simulink model "PMSMfoc_SVPWM"  (R2021b)
settings: Solver=ode3  StartTime=0.0  StopTime=0.3  FixedStep=1e-6  RelTol=1e-3
libraries: simulink x6, slpidlib x3, dsparch4 x3, spsDCVoltageSourceLib x1, spsPermanentMagnetSynchronousMachineLib x1, spsSVPWMGenerator2LevelLib x1, spsabctoAlphaBetaZeroLib x1, spsabctodq0Lib x1, spsdq0toAlphaBetaZeroLib x1, spspowerguiLib x1, spsUniversalBridgeLib x1
settings Model: Creator=zyh  LastModifiedBy=zyh
settings SolverCC: AlgebraicLoopSolver=TrustRegion
settings DataIOCC: ReturnWorkspaceOutputs=off
settings DebuggingCC: MaskedZcDiagnostic=none  IgnoredZcDiagnostic=none  SFMachineParentedDataDiag=warning  ArithmeticOperatorsInVariantConditions=warning
settings SFSimCC: CustomCodeUndefinedFunction=UseInterfaceOnly

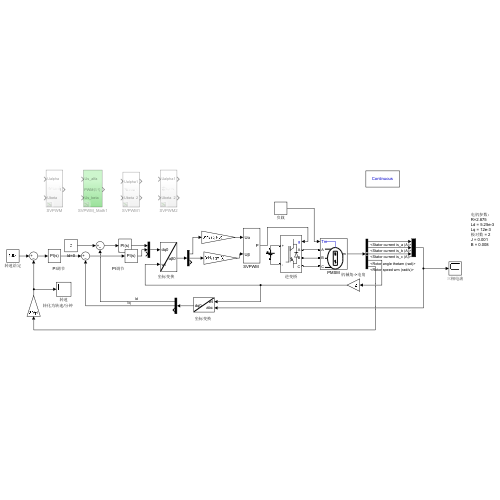
[thumbnail: Simulink's stored preview of the top-level diagram]
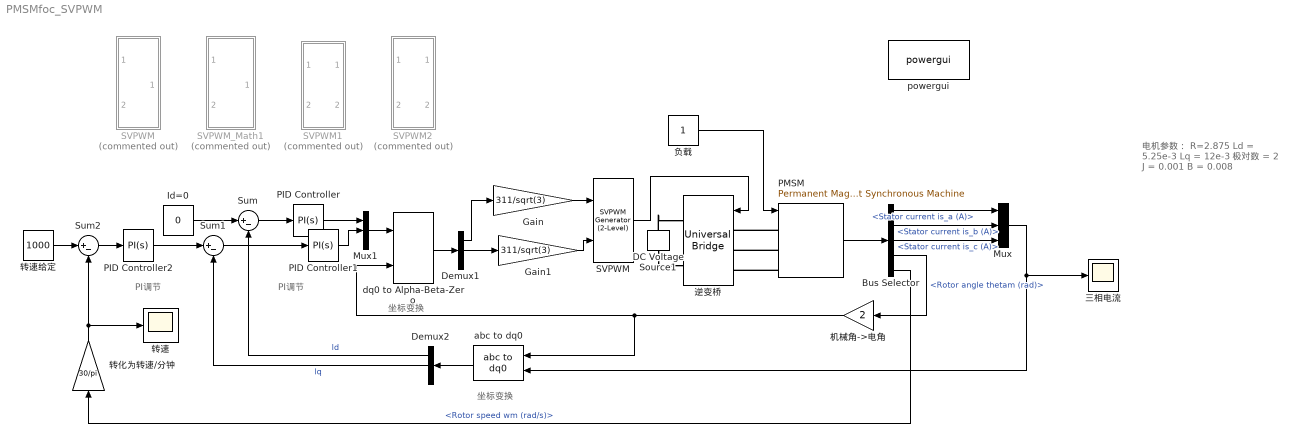
== system PMSMfoc_SVPWM ==
  note: 电机参数：
      | R=2.875
      | Ld = 5.25e-3
      | Lq = 12e-3
      | 极对数 = 2
      | J = 0.001
      | B = 0.008
  note: 坐标变换
  note: 坐标变换
  note: PI调节
  note: PI调节
  Bus Selector : BusSelector  OutputSignals=Stator current is_a (A),Stator current is_b (A),Stator current is_c (A),Rotor angle thetam (rad),Rotor speed wm (rad/s)
  DC Voltage Source1 : spsDCVoltageSourceLib/DC Voltage Source  Amplitude=311  Measurements=None
  Demux1 : Demux  Outputs=3
  Demux2 : Demux  Outputs=3
  Gain : Gain  Gain=311/sqrt(3)
  Gain1 : Gain  Gain=311/sqrt(3)
  Id=0 : Constant  Value=0
  Mux : Mux  Inputs=3
  Mux1 : Mux  Inputs=3
  PID Controller : slpidlib/PID Controller  Controller=PI  Form=Parallel  TimeDomain=Continuous-time  UseExternalTs=off  SampleTime=-1  IntegratorMethod=Forward Euler  FilterMethod=Forward Euler  ControllerParametersSource=internal  P=5  I=500  D=0  UseFilter=on  N=100  TunerSelectOption=Transfer Function Based (PID Tuner App)  InitialConditionSource=internal  InitialConditionForIntegrator=0  InitialConditionForFilter=0  DifferentiatorICPrevScaledInput=0  ExternalReset=none  TrackingMode=off  Kt=1  LimitOutput=off  SatLimitsSource=internal  UpperSaturationLimit=500  LowerSaturationLimit=-500  LinearizeAsGain=on  AntiWindupMode=none  Kb=1  POutMin=[]  POutMax=[]  IOutMin=[]  IOutMax=[]  DOutMin=[]  DOutMax=[]  NOutMin=[]  NOutMax=[]  SumOutMin=[]  SumOutMax=[]  SaturationOutMin=[]  SaturationOutMax=[]  PParamMin=[]  PParamMax=[]  IParamMin=[]  IParamMax=[]  DParamMin=[]  DParamMax=[]  NParamMin=[]  NParamMax=[]  KbParamMin=[]  KbParamMax=[]  KtParamMin=[]  KtParamMax=[]  KbOutMin=[]  KbOutMax=[]  KtOutMin=[]  KtOutMax=[]  IntegratorOutMin=[]  IntegratorOutMax=[]  FilterOutMin=[]  FilterOutMax=[]  SumI1OutMin=[]  SumI1OutMax=[]  SumI2OutMin=[]  SumI2OutMax=[]  SumI3OutMin=[]  SumI3OutMax=[]  SumI4OutMin=[]  SumI4OutMax=[]  SumDOutMin=[]  SumDOutMax=[]  DifferentiatorOutMin=[]  DifferentiatorOutMax=[]  FilterDiffOutCoefMin=[]  FilterDiffOutCoefMax=[]  ReciprocalOutMin=[]  ReciprocalOutMax=[]  SumDenOutMin=[]  SumDenOutMax=[]  SumNumOutMin=[]  SumNumOutMax=[]  DivideOutMin=[]  DivideOutMax=[]  UdiffTsProdOutMin=[]  UdiffTsProdOutMax=[]  NTsProdOutMin=[]  NTsProdOutMax=[]  UintegralTsProdOutMin=[]  UintegralTsProdOutMax=[]  UngainTsProdOutMin=[]  UngainTsProdOutMax=[]  IntegratorContinuousStateAttributes=''  IntegratorStateMustResolveToSignalObject=off  IntegratorRTWStateStorageClass=Auto  FilterContinuousStateAttributes=''  FilterStateMustResolveToSignalObject=off  FilterRTWStateStorageClass=Auto  ParallelPVariant=InternalParameters  IdealPVariant=Disabled  IVariant=InternalParameters  DVariant=Disabled  IntegratorVariant=Continuous  SatVariant=Disabled  AWVariant=Passthrough  PCopyVariant=Disabled  TRVariant=Disabled  FdbkBlocksVariant=Forward  IdealPFdbkVariant=Disabled  SatFdbkVariant=Disabled  DerivativeFilterVariant=Disabled  NVariant=Disabled  NCopyVariant=Disabled_SignalSpec  FilterICVariant=Disabled  IntegratorICVariant=InternalICs  ExternalResetVariant=Disabled  TRSumVariant=Passthrough  SumFdbkVariant=Disabled  SumVariant=Sum_PI  TsampFilterVariant=InternalTs  TsampNgainVariant=Passthrough  TsampIntegralVariant=Passthrough  ExternalSaturationOutDataTypeStr=Inherit: Same as second input
  PID Controller1 : slpidlib/PID Controller  Controller=PI  Form=Parallel  TimeDomain=Continuous-time  UseExternalTs=off  SampleTime=-1  IntegratorMethod=Forward Euler  FilterMethod=Forward Euler  ControllerParametersSource=internal  P=5  I=500  D=0  UseFilter=on  N=100  TunerSelectOption=Transfer Function Based (PID Tuner App)  InitialConditionSource=internal  InitialConditionForIntegrator=0  InitialConditionForFilter=0  DifferentiatorICPrevScaledInput=0  ExternalReset=none  TrackingMode=off  Kt=1  LimitOutput=off  SatLimitsSource=internal  UpperSaturationLimit=500  LowerSaturationLimit=-500  LinearizeAsGain=on  AntiWindupMode=none  Kb=1  POutMin=[]  POutMax=[]  IOutMin=[]  IOutMax=[]  DOutMin=[]  DOutMax=[]  NOutMin=[]  NOutMax=[]  SumOutMin=[]  SumOutMax=[]  SaturationOutMin=[]  SaturationOutMax=[]  PParamMin=[]  PParamMax=[]  IParamMin=[]  IParamMax=[]  DParamMin=[]  DParamMax=[]  NParamMin=[]  NParamMax=[]  KbParamMin=[]  KbParamMax=[]  KtParamMin=[]  KtParamMax=[]  KbOutMin=[]  KbOutMax=[]  KtOutMin=[]  KtOutMax=[]  IntegratorOutMin=[]  IntegratorOutMax=[]  FilterOutMin=[]  FilterOutMax=[]  SumI1OutMin=[]  SumI1OutMax=[]  SumI2OutMin=[]  SumI2OutMax=[]  SumI3OutMin=[]  SumI3OutMax=[]  SumI4OutMin=[]  SumI4OutMax=[]  SumDOutMin=[]  SumDOutMax=[]  DifferentiatorOutMin=[]  DifferentiatorOutMax=[]  FilterDiffOutCoefMin=[]  FilterDiffOutCoefMax=[]  ReciprocalOutMin=[]  ReciprocalOutMax=[]  SumDenOutMin=[]  SumDenOutMax=[]  SumNumOutMin=[]  SumNumOutMax=[]  DivideOutMin=[]  DivideOutMax=[]  UdiffTsProdOutMin=[]  UdiffTsProdOutMax=[]  NTsProdOutMin=[]  NTsProdOutMax=[]  UintegralTsProdOutMin=[]  UintegralTsProdOutMax=[]  UngainTsProdOutMin=[]  UngainTsProdOutMax=[]  IntegratorContinuousStateAttributes=''  IntegratorStateMustResolveToSignalObject=off  IntegratorRTWStateStorageClass=Auto  FilterContinuousStateAttributes=''  FilterStateMustResolveToSignalObject=off  FilterRTWStateStorageClass=Auto  ParallelPVariant=InternalParameters  IdealPVariant=Disabled  IVariant=InternalParameters  DVariant=Disabled  IntegratorVariant=Continuous  SatVariant=Disabled  AWVariant=Passthrough  PCopyVariant=Disabled  TRVariant=Disabled  FdbkBlocksVariant=Forward  IdealPFdbkVariant=Disabled  SatFdbkVariant=Disabled  DerivativeFilterVariant=Disabled  NVariant=Disabled  NCopyVariant=Disabled_SignalSpec  FilterICVariant=Disabled  IntegratorICVariant=InternalICs  ExternalResetVariant=Disabled  TRSumVariant=Passthrough  SumFdbkVariant=Disabled  SumVariant=Sum_PI  TsampFilterVariant=InternalTs  TsampNgainVariant=Passthrough  TsampIntegralVariant=Passthrough  ExternalSaturationOutDataTypeStr=Inherit: Same as second input
  PID Controller2 : slpidlib/PID Controller  Controller=PI  Form=Parallel  TimeDomain=Continuous-time  UseExternalTs=off  SampleTime=-1  IntegratorMethod=Forward Euler  FilterMethod=Forward Euler  ControllerParametersSource=internal  P=0.1  I=3  D=0  UseFilter=on  N=100  TunerSelectOption=Transfer Function Based (PID Tuner App)  InitialConditionSource=internal  InitialConditionForIntegrator=0  InitialConditionForFilter=0  DifferentiatorICPrevScaledInput=0  ExternalReset=none  TrackingMode=off  Kt=1  LimitOutput=off  SatLimitsSource=internal  UpperSaturationLimit=30  LowerSaturationLimit=-30  LinearizeAsGain=on  AntiWindupMode=none  Kb=1  POutMin=[]  POutMax=[]  IOutMin=[]  IOutMax=[]  DOutMin=[]  DOutMax=[]  NOutMin=[]  NOutMax=[]  SumOutMin=[]  SumOutMax=[]  SaturationOutMin=[]  SaturationOutMax=[]  PParamMin=[]  PParamMax=[]  IParamMin=[]  IParamMax=[]  DParamMin=[]  DParamMax=[]  NParamMin=[]  NParamMax=[]  KbParamMin=[]  KbParamMax=[]  KtParamMin=[]  KtParamMax=[]  KbOutMin=[]  KbOutMax=[]  KtOutMin=[]  KtOutMax=[]  IntegratorOutMin=[]  IntegratorOutMax=[]  FilterOutMin=[]  FilterOutMax=[]  SumI1OutMin=[]  SumI1OutMax=[]  SumI2OutMin=[]  SumI2OutMax=[]  SumI3OutMin=[]  SumI3OutMax=[]  SumI4OutMin=[]  SumI4OutMax=[]  SumDOutMin=[]  SumDOutMax=[]  DifferentiatorOutMin=[]  DifferentiatorOutMax=[]  FilterDiffOutCoefMin=[]  FilterDiffOutCoefMax=[]  ReciprocalOutMin=[]  ReciprocalOutMax=[]  SumDenOutMin=[]  SumDenOutMax=[]  SumNumOutMin=[]  SumNumOutMax=[]  DivideOutMin=[]  DivideOutMax=[]  UdiffTsProdOutMin=[]  UdiffTsProdOutMax=[]  NTsProdOutMin=[]  NTsProdOutMax=[]  UintegralTsProdOutMin=[]  UintegralTsProdOutMax=[]  UngainTsProdOutMin=[]  UngainTsProdOutMax=[]  IntegratorContinuousStateAttributes=''  IntegratorStateMustResolveToSignalObject=off  IntegratorRTWStateStorageClass=Auto  FilterContinuousStateAttributes=''  FilterStateMustResolveToSignalObject=off  FilterRTWStateStorageClass=Auto  ParallelPVariant=InternalParameters  IdealPVariant=Disabled  IVariant=InternalParameters  DVariant=Disabled  IntegratorVariant=Continuous  SatVariant=Disabled  AWVariant=Passthrough  PCopyVariant=Disabled  TRVariant=Disabled  FdbkBlocksVariant=Forward  IdealPFdbkVariant=Disabled  SatFdbkVariant=Disabled  DerivativeFilterVariant=Disabled  NVariant=Disabled  NCopyVariant=Disabled_SignalSpec  FilterICVariant=Disabled  IntegratorICVariant=InternalICs  ExternalResetVariant=Disabled  TRSumVariant=Passthrough  SumFdbkVariant=Disabled  SumVariant=Sum_PI  TsampFilterVariant=InternalTs  TsampNgainVariant=Passthrough  TsampIntegralVariant=Passthrough  ExternalSaturationOutDataTypeStr=Inherit: Same as second input
  PMSM : spsPermanentMagnetSynchronousMachineLib/Permanent Magnet Synchronous Machine  NbPhases=3  FluxDistribution=Sinusoidal  RotorType=Salient-pole  MechanicalLoad=Torque Tm  PresetModel=No  ShowDetailedParameters=on  MeasurementBus=off  Resistance=2.875  Inductance=8.5e-3  dqInductances=[5.25e-3 12e-3]  La=8.5e-3  MachineConstant=Flux linkage established by magnets (V.s)  Flux=0.175  VoltageCst=63.483  TorqueCst=0.525  Flat=120  Mechanical=[0.001 0.008 2 0]  PolePairs=2  InitialConditions=[0,0, 0,0]  InitialConditions5ph=[0 0 0 0 0 0]  RefAngle=Aligned with phase A axis (original Park)  IterativeDiscreteModel=Trapezoidal non iterative  TsBlock=-1  TsPowergui=0
  SVPWM : Subsystem  Commented=on
  "SVPWM " : spsSVPWMGenerator2LevelLib/SVPWM Generator (2-Level)  InputType=alpha-beta components  SwitchingPattern=Pattern #1  Fc=5000  ParUref=[0.8 -30 50]  Ts=0
      settings: SourceProductBaseCode=PS
  SVPWM1 : Subsystem  Commented=on
  SVPWM2 : Subsystem  Commented=on
  SVPWM_Math1 : Subsystem  Commented=on
  Sum : Sum  Inputs=|+-
  Sum1 : Sum  Inputs=|+-
  Sum2 : Sum  Inputs=|+-
  abc to dq0 : spsabctodq0Lib/abc to dq0  Alignment=Aligned with phase A axis
  dq0 to Alpha-Beta-Zero : spsdq0toAlphaBetaZeroLib/dq0 to Alpha-Beta-Zero  Alignment=Aligned with phase A axis
      settings: SourceProductBaseCode=PS
  powergui : spspowerguiLib/powergui  Priority=1  SimulationMode=Continuous  SampleTime=1e-6  frequency=60  Iterations=50  frequencyindice=0  Pbase=100e6  ErrMax=1e-4  UnitsV=kV  UnitsW=MW  buscounter=0  FunctionMessages=off  echomessages=off  EnableUseOfTLC=off  CurrentSourceSwitches=off  DisableSnubberDevices=off  DisableRonSwitches=off  DisableVfSwitches=off  DisplayEquations=off  AutomaticDiscreteSolvers=off  SolverType=Tustin/Backward Euler (TBE)  Interpol=off  ExternalGateDelay=off  methode=off  Ts=100  x0status=blocks  SPID=on  SwTol=0  HookPort=off  NonlinearTolerance=1e-4  nMaxIteration=100  ContinueOnMaxIteration=off  RestoreLinks=warning  ResistiveCurrentMeasurement=off  Frange=[0:2:500]  Ylog=off  Xlog=on  ShowGrid=off  save=off  variable=ZData  structure=0  ZoomFFT=off  StartTime=0.0  cycles=1  DisplayStyle=1  fundamental=60  FreqAxis=off  MaxFrequency=1000  frequencyindicesteady=1  RmsSteady=1  display=off
  三相电流 : Scope
  机械角->电角 : Gain  Gain=2
  负载 : Constant
  转化为转速/分钟 : Gain  Gain=30/pi
  转速 : Scope
  转速给定 : Constant  Value=1000
  逆变桥 : spsUniversalBridgeLib/Universal Bridge  Arms=3  SnubberResistance=1e5  SnubberCapacitance=inf  Device=IGBT / Diodes  Ron=1e-3  Lon=0  ForwardVoltages="[  0  0  ]"  ForwardVoltage=0  GTOparameters=[ 10e-6 , 20e-6 ]  IGBTparameters=[ 1e-6 , 2e-6 ]  Measurements=None  Measurements_2=None  converterType=Rectifier
  wires:
  Id=0/1 -> Sum/1
  Bus Selector/1 -> Mux/1  "<Stator current is_a (A)>"
  Bus Selector/2 -> Mux/2  "<Stator current is_b (A)>"
  Bus Selector/3 -> Mux/3  "<Stator current is_c (A)>"
  Mux/1 -> abc to dq0/1, 三相电流/1
  Bus Selector/5 -> 转化为转速/分钟/1  "<Rotor speed wm (rad/s)>"
  Bus Selector/4 -> 机械角->电角/1  "<Rotor angle thetam (rad)>"
  机械角->电角/1 -> abc to dq0/2, dq0 to Alpha-Beta-Zero/2
  Demux2/1 -> Sum/2  "ld"
  Demux2/2 -> Sum1/2  "lq"
  Sum/1 -> PID Controller/1
  PID Controller/1 -> Mux1/1
  PID Controller1/1 -> Mux1/2
  Sum1/1 -> PID Controller1/1
  转速给定/1 -> Sum2/1
  转化为转速/分钟/1 -> 转速/1, Sum2/2
  Sum2/1 -> PID Controller2/1
  Mux1/1 -> dq0 to Alpha-Beta-Zero/1
  PID Controller2/1 -> Sum1/1
  Demux1/1 -> Gain/1
  PMSM/1 -> Bus Selector/1
  dq0 to Alpha-Beta-Zero/1 -> Demux1/1
  Demux1/2 -> Gain1/1
  abc to dq0/1 -> Demux2/1
  负载/1 -> PMSM/1
  "SVPWM "/1 -> 逆变桥/1
  Gain/1 -> "SVPWM "/1
  Gain1/1 -> "SVPWM "/2
  connections:
  PMSM/LConn1 -- 逆变桥/LConn1
  PMSM/LConn2 -- 逆变桥/LConn2
  DC Voltage Source1/RConn1 -- 逆变桥/RConn1
  DC Voltage Source1/LConn1 -- 逆变桥/RConn2
  PMSM/LConn3 -- 逆变桥/LConn3

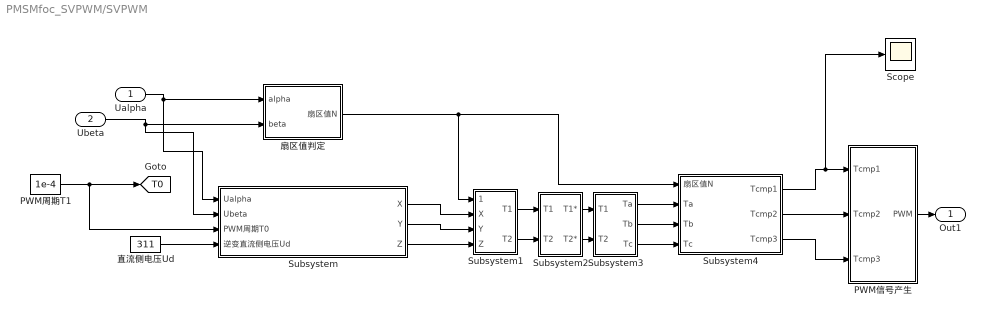
== system PMSMfoc_SVPWM/SVPWM ==
  Ualpha : Inport
  Ubeta : Inport  Port=2
  PWM信号产生 : Subsystem
  PWM周期T1 : Constant  Value=1e-4
  Scope : Scope
  Subsystem : Subsystem
  Subsystem1 : Subsystem
  Subsystem2 : Subsystem
  Subsystem3 : Subsystem
  Subsystem4 : Subsystem
  扇区值判定 : Subsystem
  直流侧电压Ud : Constant  Value=311
  Out1 : Outport  VectorParamsAs1DForOutWhenUnconnected=off
  tag scope: T0=global
  wires:
  Subsystem2/2(T2*) -> Subsystem3/2(T2)
  Subsystem1/2(T2) -> Subsystem2/2(T2)
  Subsystem4/1(Tcmp1) -> PWM信号产生/1(Tcmp1), Scope/1
  Subsystem3/2(Tb) -> Subsystem4/3(Tb)
  直流侧电压Ud/1 -> Subsystem/4(逆变直流侧电压Ud)
  Ualpha/1 -> 扇区值判定/1(alpha), Subsystem/1(Ualpha)
  Subsystem/3(Z) -> Subsystem1/4(Z)
  Subsystem3/3(Tc) -> Subsystem4/4(Tc)
  PWM信号产生/1(PWM) -> Out1/1
  Subsystem3/1(Ta) -> Subsystem4/2(Ta)
  PWM周期T1/1 -> Subsystem/3(PWM周期T0), [T0]
  Subsystem4/2(Tcmp2) -> PWM信号产生/2(Tcmp2)
  扇区值判定/1(扇区值N) -> Subsystem4/1(扇区值N), Subsystem1/1(扇区值N)
  Subsystem4/3(Tcmp3) -> PWM信号产生/3(Tcmp3)
  Subsystem/2(Y) -> Subsystem1/3(Y)
  Ubeta/1 -> 扇区值判定/2(beta), Subsystem/2(Ubeta)
  Subsystem/1(X) -> Subsystem1/2(X)
  Subsystem1/1(T1) -> Subsystem2/1(T1)
  Subsystem2/1(T1*) -> Subsystem3/1(T1)

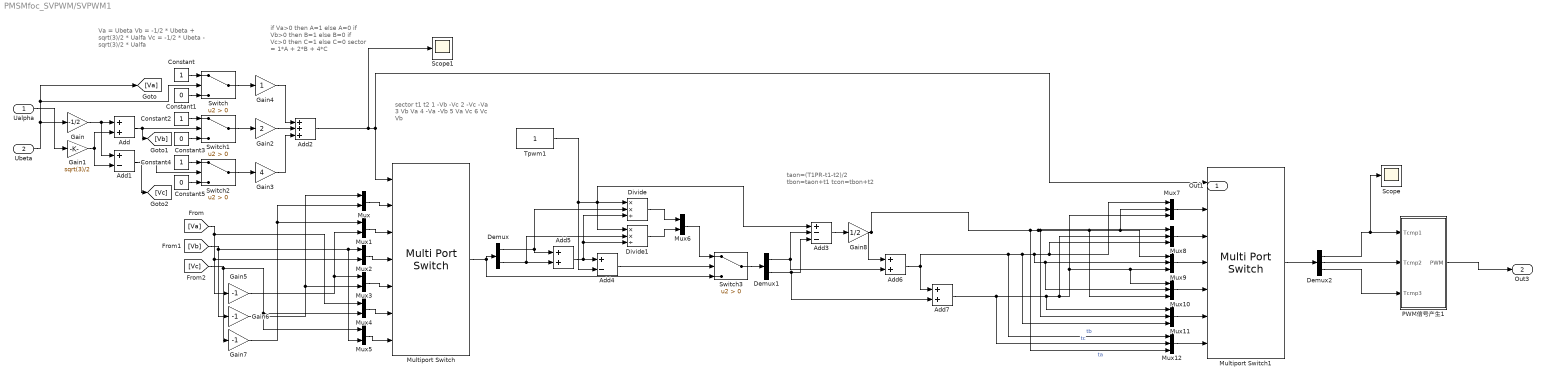
== system PMSMfoc_SVPWM/SVPWM1 ==
  note: taon=(T1PR-t1-t2)/2
      | tbon=taon+t1
      | tcon=tbon+t2
  note: sector   t1       t2
      | 1        -Vb     -Vc
      | 2        -Vc     -Va
      | 3         Vb      Va
      | 4        -Va     -Vb
      | 5         Va      Vc
      | 6         Vc      Vb
  note: if Va>0 then A=1 else A=0
      | if Vb>0 then B=1 else B=0
      | if Vc>0 then C=1 else C=0
      | sector = 1*A + 2*B + 4*C
  note: Va = Ubeta
      | Vb = -1/2 * Ubeta + sqrt(3)/2 * Ualfa
      | Vc = -1/2 * Ubeta - sqrt(3)/2 * Ualfa
  Ualpha : Inport
  Ubeta : Inport  Port=2
  Add{,5..7} (4 alike) : Sum
  Add1 : Sum  Inputs=+-
  Add2 : Sum  Inputs=+++
  Add3 : Sum  Inputs=+--
  Add4 : Sum  Inputs=+-
  Constant : Constant
  Constant1 : Constant  Value=0
  Constant2 : Constant
  Constant3 : Constant  Value=0
  Constant4 : Constant
  Constant5 : Constant  Value=0
  Demux : Demux  Outputs=2
  Demux1 : Demux  Outputs=2
  Demux2 : Demux  Outputs=3
  Divide : Product  Inputs=**/
  Divide1 : Product  Inputs=**/
  Gain : Gain  Gain=-1/2
  Gain1 : Gain  Gain=sqrt(3)/2
  Gain2 : Gain  Gain=2
  Gain3 : Gain  Gain=4
  Gain4 : Gain
  Gain5 : Gain  Gain=-1
  Gain6 : Gain  Gain=-1
  Gain7 : Gain  Gain=-1
  Gain8 : Gain  Gain=1/2
  Multiport Switch : MultiPortSwitch  Inputs=6  DiagnosticForDefault=None  OutDataTypeStr=double
  Multiport Switch1 : MultiPortSwitch  Inputs=6  DiagnosticForDefault=None  OutDataTypeStr=double
  Mux{,1..6} (7 alike) : Mux  Inputs=2
  Mux{7..12} (6 alike) : Mux  Inputs=3
  PWM信号产生1 : Subsystem
  Scope : Scope
  Scope1 : Scope
  Switch{,1..3} (4 alike) : Switch  Criteria=u2 > Threshold
  Tpwm1 : Constant
  Out1 : Outport  VectorParamsAs1DForOutWhenUnconnected=off
  Out3 : Outport  Port=2  VectorParamsAs1DForOutWhenUnconnected=off
  wires:
  Ualpha/1 -> Gain1/1
  Ubeta/1 -> Gain/1, Switch/2, [Va]
  Gain/1 -> Add1/1, Add/1
  Gain1/1 -> Add/2, Add1/2
  Add1/1 -> [Vc], Switch2/2
  Constant/1 -> Switch/1
  Constant1/1 -> Switch/3
  Constant3/1 -> Switch1/3
  Constant2/1 -> Switch1/1
  Add/1 -> [Vb], Switch1/2
  Constant4/1 -> Switch2/1
  Constant5/1 -> Switch2/3
  Switch1/1 -> Gain2/1
  Switch2/1 -> Gain3/1
  Switch/1 -> Gain4/1
  Gain4/1 -> Add2/1
  Gain2/1 -> Add2/2
  Gain3/1 -> Add2/3
  Add2/1 -> Scope1/1, Multiport Switch/1, Multiport Switch1/1
  [Va] -> Mux4/1, Mux2/2, Gain5/1
  [Vb] -> Mux5/2, Mux2/1, Gain6/1
  [Vc] -> Mux5/1, Mux4/2, Gain7/1
  Mux/1 -> Multiport Switch/2
  Gain6/1 -> Mux3/2, Mux/1
  Gain7/1 -> Mux/2, Mux1/1
  Gain5/1 -> Mux3/1, Mux1/2
  Mux1/1 -> Multiport Switch/3
  Mux2/1 -> Multiport Switch/4
  Mux3/1 -> Multiport Switch/5
  Mux4/1 -> Multiport Switch/6
  Mux5/1 -> Multiport Switch/7
  Multiport Switch/1 -> Demux/1, Switch3/3
  Demux/1 -> Add5/1, Divide/2
  Demux/2 -> Divide1/2, Add5/2
  Add5/1 -> Divide1/3, Divide/3, Add4/1
  Tpwm1/1 -> Add4/2, Add3/1, Divide1/1, Divide/1
  Add4/1 -> Switch3/2
  Divide/1 -> Mux6/1
  Divide1/1 -> Mux6/2
  Mux6/1 -> Switch3/1
  Switch3/1 -> Demux1/1
  Demux1/1 -> Add3/2, Add6/2
  Demux1/2 -> Add7/2, Add3/3
  Add3/1 -> Gain8/1
  Gain8/1 -> Mux12/3, Mux11/2, Mux10/3, Mux9/1, Mux7/2, Mux8/1, Add6/1  "ta"
  Add6/1 -> Mux12/1, Mux11/3, Mux10/2, Mux9/2, Mux8/3, Mux7/1, Add7/1  "tb"
  Add7/1 -> Mux12/2, Mux11/1, Mux8/2, Mux10/1, Mux9/3, Mux7/3  "tc"
  PWM信号产生1/1(PWM) -> Out3/1
  Mux7/1 -> Multiport Switch1/2
  Mux8/1 -> Multiport Switch1/3
  Mux9/1 -> Multiport Switch1/4
  Mux10/1 -> Multiport Switch1/5
  Mux11/1 -> Multiport Switch1/6
  Mux12/1 -> Multiport Switch1/7
  Multiport Switch1/1 -> Demux2/1
  Demux2/1 -> Scope/1, PWM信号产生1/1(Tcmp1)
  Demux2/2 -> PWM信号产生1/2(Tcmp2)
  Demux2/3 -> PWM信号产生1/3(Tcmp3)

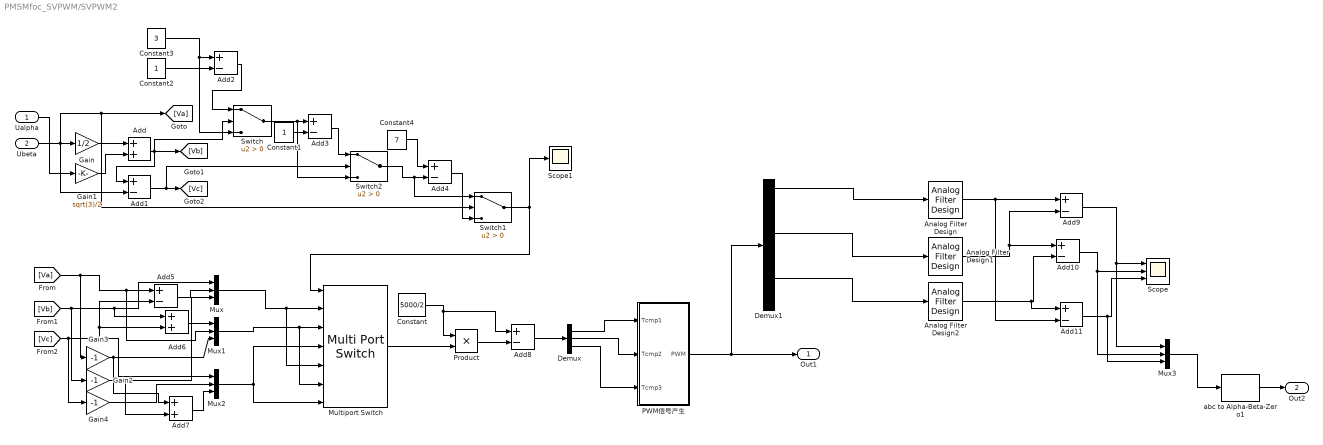
== system PMSMfoc_SVPWM/SVPWM2 ==
  Ualpha : Inport
  Ubeta : Inport  Port=2
  Add : Sum
  Add{1..5,8..11} (9 alike) : Sum  Inputs=+-
  Add6 : Sum
  Add7 : Sum
  Analog Filter Design : dsparch4/Analog Filter Design  method=Butterworth  filttype=Lowpass  N=2  Wlo=10000  Whi=80  Rp=2  Rs=40
  Analog Filter Design1 : dsparch4/Analog Filter Design  method=Butterworth  filttype=Lowpass  N=2  Wlo=10000  Whi=80  Rp=2  Rs=40
  Analog Filter Design2 : dsparch4/Analog Filter Design  method=Butterworth  filttype=Lowpass  N=2  Wlo=10000  Whi=80  Rp=2  Rs=40
  Constant : Constant  Value=5000/2
  Constant1 : Constant
  Constant2 : Constant
  Constant3 : Constant  Value=3
  Constant4 : Constant  Value=7
  Demux : Demux  Outputs=3
  Demux1 : Demux  Outputs=6
  Gain : Gain  Gain=1/2
  Gain1 : Gain  Gain=sqrt(3)/2
  Gain2 : Gain  Gain=-1
  Gain3 : Gain  Gain=-1
  Gain4 : Gain  Gain=-1
  Multiport Switch : MultiPortSwitch  Inputs=6  DiagnosticForDefault=None  OutDataTypeStr=double
  Mux{,1..3} (4 alike) : Mux  Inputs=3
  PWM信号产生 : Subsystem
  Product : Product
  Scope : Scope  NumInputPorts=3
  Scope1 : Scope
  Switch : Switch  Criteria=u2 > Threshold
  Switch1 : Switch  Criteria=u2 > Threshold
  Switch2 : Switch  Criteria=u2 > Threshold
  abc to Alpha-Beta-Zero1 : spsabctoAlphaBetaZeroLib/abc to Alpha-Beta-Zero
      settings: SourceProductBaseCode=PS
  Out1 : Outport  VectorParamsAs1DForOutWhenUnconnected=off
  Out2 : Outport  Port=2
  wires:
  PWM信号产生/1(PWM) -> Demux1/1, Out1/1
  Ualpha/1 -> Gain1/1
  Gain/1 -> Add/1
  Add/1 -> Switch/2, Add1/1, [Vb]
  Gain1/1 -> Add/2
  Ubeta/1 -> Add1/2, Gain/1, [Va], Switch1/2
  Add2/1 -> Switch/1
  Constant3/1 -> Switch/3, Add2/1
  Add1/1 -> Switch2/2, [Vc]
  Switch/1 -> Switch2/3, Add3/1
  Constant2/1 -> Add2/2
  Constant1/1 -> Add3/2
  Add3/1 -> Switch2/1
  Constant4/1 -> Add4/1
  Switch2/1 -> Switch1/1, Add4/2
  [Vb] -> Gain2/1, Add6/1, Mux/1
  [Va] -> Gain3/1, Mux1/2, Add5/1
  [Vc] -> Gain4/1, Mux2/1, Add6/2, Add5/2
  Add5/1 -> Mux/2
  Gain2/1 -> Add7/2, Mux/3
  Add6/1 -> Mux1/1
  Gain3/1 -> Add7/1, Mux1/3
  Gain4/1 -> Mux2/2
  Add7/1 -> Mux2/3
  Mux/1 -> Multiport Switch/5, Multiport Switch/2
  Mux1/1 -> Multiport Switch/6, Multiport Switch/3
  Mux2/1 -> Multiport Switch/4, Multiport Switch/7
  Constant/1 -> Add8/1, Product/1
  Multiport Switch/1 -> Product/2
  Add8/1 -> Demux/1
  Demux/1 -> PWM信号产生/1(Tcmp1)
  Demux/2 -> PWM信号产生/2(Tcmp2)
  Demux/3 -> PWM信号产生/3(Tcmp3)
  Switch1/1 -> Multiport Switch/1, Scope1/1
  Add4/1 -> Switch1/3
  Product/1 -> Add8/2
  Demux1/1 -> Analog Filter Design/1
  Demux1/3 -> Analog Filter Design1/1
  Demux1/5 -> Analog Filter Design2/1
  Analog Filter Design/1 -> Add11/2, Add9/1
  Analog Filter Design1/1 -> Add10/1, Add9/2
  Analog Filter Design2/1 -> Add11/1, Add10/2
  Add9/1 -> Mux3/1, Scope/1
  Add10/1 -> Mux3/2, Scope/2
  Add11/1 -> Mux3/3, Scope/3
  Mux3/1 -> abc to Alpha-Beta-Zero1/1
  abc to Alpha-Beta-Zero1/1 -> Out2/1

== system PMSMfoc_SVPWM/SVPWM_Math1 ==
  Us_alfa : Inport
  Us_beta : Inport  Port=2
  Clock1 : Clock
  PWM : MATLAB Function  TreatAsAtomicUnit=on
  作用时间计算 : MATLAB Function  TreatAsAtomicUnit=on
  开关频率 : Constant  Value=0.0001
  直流侧电压Ud : Constant  Value=311
  采样周期 : Constant  Value=0.00001
  PWM信号 : Outport  VectorParamsAs1DForOutWhenUnconnected=off
  wires:
  作用时间计算/1(S) -> PWM/1(S)
  Clock1/1 -> PWM/4(time)
  开关频率/1 -> 作用时间计算/4(T0)
  直流侧电压Ud/1 -> 作用时间计算/3(Udc)
  Us_beta/1 -> 作用时间计算/2(Us_beta)
  Us_alfa/1 -> 作用时间计算/1(Us_alfa)
  PWM/1(PWM) -> PWM信号/1
  作用时间计算/3(t2) -> PWM/3(t2)
  作用时间计算/2(t1) -> PWM/2(t1)
  采样周期/1 -> PWM/5(T0)

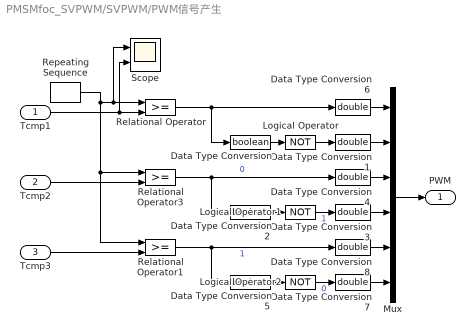
== system PMSMfoc_SVPWM/SVPWM/PWM信号产生 ==
  Tcmp1 : Inport
  Tcmp2 : Inport  Port=2
  Tcmp3 : Inport  Port=3
  Data Type Conversion : DataTypeConversion  OutDataTypeStr=boolean
  Data Type Conversion{1,3..4,6..8} (6 alike) : DataTypeConversion  OutDataTypeStr=double
  Data Type Conversion2 : DataTypeConversion  OutDataTypeStr=boolean
  Data Type Conversion5 : DataTypeConversion  OutDataTypeStr=boolean
  Logical Operator : Logic  Operator=NOT  AllPortsSameDT=off  OutDataTypeStr=boolean
  Logical Operator1 : Logic  Operator=NOT  AllPortsSameDT=off  OutDataTypeStr=boolean
  Logical Operator2 : Logic  Operator=NOT  AllPortsSameDT=off  OutDataTypeStr=boolean
  Mux : Mux  Inputs=6
  Relational Operator : RelationalOperator  OutDataTypeStr=boolean  RndMeth=Nearest
  Relational Operator1 : RelationalOperator  OutDataTypeStr=boolean  RndMeth=Nearest
  Relational Operator3 : RelationalOperator  OutDataTypeStr=boolean  RndMeth=Nearest
  Repeating Sequence : simulink/Sources/Repeating Sequence  rep_seq_t=[0 1e-4 2e-4]  rep_seq_y=[0 0.5e-4 0]
  Scope : Scope  NumInputPorts=2
  PWM : Outport  VectorParamsAs1DForOutWhenUnconnected=off
  wires:
  Data Type Conversion6/1 -> Mux/1
  Mux/1 -> PWM/1
  Data Type Conversion7/1 -> Mux/6
  Data Type Conversion8/1 -> Mux/5
  Data Type Conversion3/1 -> Mux/4
  Data Type Conversion4/1 -> Mux/3
  Data Type Conversion1/1 -> Mux/2
  Tcmp3/1 -> Relational Operator1/2
  Tcmp2/1 -> Relational Operator3/2
  Tcmp1/1 -> Relational Operator/2, Scope/2
  Repeating Sequence/1 -> Relational Operator/1, Scope/1, Relational Operator3/1, Relational Operator1/1
  Logical Operator2/1 -> Data Type Conversion7/1  "0"
  Data Type Conversion5/1 -> Logical Operator2/1
  Relational Operator1/1 -> Data Type Conversion5/1, Data Type Conversion8/1  "1"
  Data Type Conversion2/1 -> Logical Operator1/1
  Relational Operator3/1 -> Data Type Conversion2/1, Data Type Conversion4/1  "0"
  Logical Operator1/1 -> Data Type Conversion3/1  "1"
  Relational Operator/1 -> Data Type Conversion/1, Data Type Conversion6/1
  Logical Operator/1 -> Data Type Conversion1/1
  Data Type Conversion/1 -> Logical Operator/1

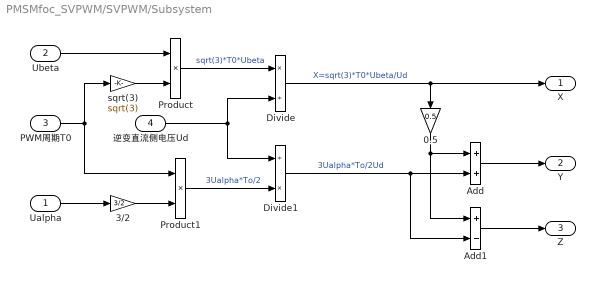
== system PMSMfoc_SVPWM/SVPWM/Subsystem ==
  Ualpha : Inport
  Ubeta : Inport  Port=2
  PWM周期T0 : Inport  Port=3
  逆变直流侧电压Ud : Inport  Port=4
  0.5 : Gain  Gain=0.5
  3/2 : Gain  Gain=3/2
  Add : Sum
  Add1 : Sum  Inputs=+-
  Divide : Product  Inputs=*/
  Divide1 : Product  Inputs=/*
  Product : Product
  Product1 : Product
  "sqrt(3) " : Gain  Gain=sqrt(3)
  X : Outport  VectorParamsAs1DForOutWhenUnconnected=off
  Y : Outport  Port=2  VectorParamsAs1DForOutWhenUnconnected=off
  Z : Outport  Port=3  VectorParamsAs1DForOutWhenUnconnected=off
  wires:
  Product/1 -> Divide/1  "sqrt(3)*T0*Ubeta"
  Add1/1 -> Z/1
  Divide1/1 -> Add/2, Add1/2  "3Ualpha*To/2Ud"
  Ubeta/1 -> Product/1
  Ualpha/1 -> 3/2/1
  Add/1 -> Y/1
  Product1/1 -> Divide1/2  "3Ualpha*To/2"
  3/2/1 -> Product1/2
  "sqrt(3) "/1 -> Product/2
  PWM周期T0/1 -> Product1/1, "sqrt(3) "/1
  0.5/1 -> Add1/1, Add/1
  逆变直流侧电压Ud/1 -> Divide/2, Divide1/1
  Divide/1 -> 0.5/1, X/1  "X=sqrt(3)*T0*Ubeta/Ud"

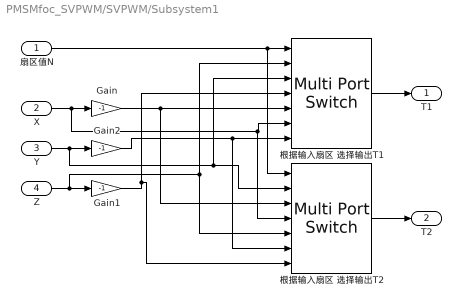
== system PMSMfoc_SVPWM/SVPWM/Subsystem1 ==
  扇区值N : Inport
  X : Inport  Port=2
  Y : Inport  Port=3
  Z : Inport  Port=4
  Gain : Gain  Gain=-1
  Gain1 : Gain  Gain=-1
  Gain2 : Gain  Gain=-1
  根据输入扇区 选择输出T1 : MultiPortSwitch  Inputs=6  DiagnosticForDefault=None
  根据输入扇区 选择输出T2 : MultiPortSwitch  Inputs=6  DiagnosticForDefault=None
  T1 : Outport  VectorParamsAs1DForOutWhenUnconnected=off
  T2 : Outport  Port=2  VectorParamsAs1DForOutWhenUnconnected=off
  wires:
  扇区值N/1 -> 根据输入扇区 选择输出T1/1, 根据输入扇区 选择输出T2/1
  Gain2/1 -> 根据输入扇区 选择输出T1/7, 根据输入扇区 选择输出T2/6
  根据输入扇区 选择输出T2/1 -> T2/1
  根据输入扇区 选择输出T1/1 -> T1/1
  Gain/1 -> 根据输入扇区 选择输出T2/3, 根据输入扇区 选择输出T1/5
  Gain1/1 -> 根据输入扇区 选择输出T1/4, 根据输入扇区 选择输出T2/7
  Z/1 -> Gain1/1, 根据输入扇区 选择输出T1/2, 根据输入扇区 选择输出T2/5
  Y/1 -> Gain2/1, 根据输入扇区 选择输出T2/2, 根据输入扇区 选择输出T1/3
  X/1 -> Gain/1, 根据输入扇区 选择输出T1/6, 根据输入扇区 选择输出T2/4

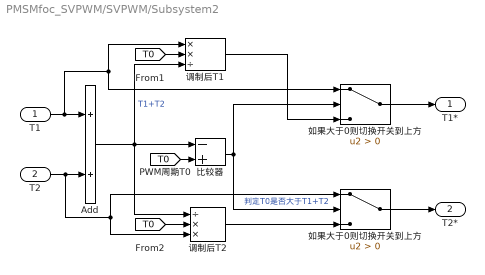
== system PMSMfoc_SVPWM/SVPWM/Subsystem2 ==
  T1 : Inport
  T2 : Inport  Port=2
  Add : Sum
  如果大于0则切换开关到上方 : Switch  Criteria=u2 > Threshold
  "如果大于0则切换开关到上方 " : Switch  Criteria=u2 > Threshold
  比较器 : Sum  Inputs=-+
  调制后T1 : Product  Inputs=**/
  调制后T2 : Product  Inputs=/**
  T1* : Outport  VectorParamsAs1DForOutWhenUnconnected=off
  T2* : Outport  Port=2  VectorParamsAs1DForOutWhenUnconnected=off
  wires:
  T2/1 -> Add/2, 调制后T2/3, "如果大于0则切换开关到上方 "/1
  调制后T2/1 -> "如果大于0则切换开关到上方 "/3
  如果大于0则切换开关到上方/1 -> T1*/1
  [T0] -> 比较器/2
  T1/1 -> Add/1, 调制后T1/1, 如果大于0则切换开关到上方/1
  [T0] -> 调制后T1/2
  Add/1 -> 调制后T1/3, 比较器/1, 调制后T2/1  "T1+T2"
  [T0] -> 调制后T2/2
  比较器/1 -> 如果大于0则切换开关到上方/2, "如果大于0则切换开关到上方 "/2  "判定T0是否大于T1+T2"
  "如果大于0则切换开关到上方 "/1 -> T2*/1
  调制后T1/1 -> 如果大于0则切换开关到上方/3

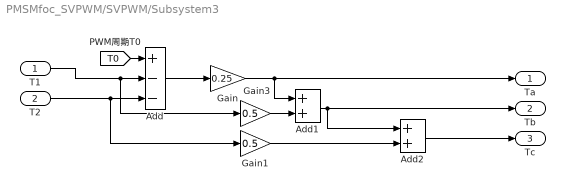
== system PMSMfoc_SVPWM/SVPWM/Subsystem3 ==
  T1 : Inport
  T2 : Inport  Port=2
  Add : Sum  Inputs=+--
  Add1 : Sum
  Add2 : Sum
  Gain : Gain  Gain=0.25
  Gain1 : Gain  Gain=0.5
  Gain3 : Gain  Gain=0.5
  Ta : Outport  VectorParamsAs1DForOutWhenUnconnected=off
  Tb : Outport  Port=2  VectorParamsAs1DForOutWhenUnconnected=off
  Tc : Outport  Port=3  VectorParamsAs1DForOutWhenUnconnected=off
  wires:
  T2/1 -> Add/3, Gain1/1
  Gain/1 -> Add1/1, Ta/1
  Gain1/1 -> Add2/2
  Gain3/1 -> Add1/2
  Add1/1 -> Add2/1, Tb/1
  T1/1 -> Add/2, Gain3/1
  [T0] -> Add/1
  Add/1 -> Gain/1
  Add2/1 -> Tc/1

== system PMSMfoc_SVPWM/SVPWM/Subsystem4 ==
  扇区值N : Inport
  Ta : Inport  Port=2
  Tb : Inport  Port=3
  Tc : Inport  Port=4
  Multiport Switch : MultiPortSwitch  Inputs=6  DiagnosticForDefault=None  OutDataTypeStr=double
  Multiport Switch1 : MultiPortSwitch  Inputs=6  DiagnosticForDefault=None  OutDataTypeStr=double
  Multiport Switch2 : MultiPortSwitch  Inputs=6  DiagnosticForDefault=None  OutDataTypeStr=double
  Tcmp1 : Outport  VectorParamsAs1DForOutWhenUnconnected=off
  Tcmp2 : Outport  Port=2  VectorParamsAs1DForOutWhenUnconnected=off
  Tcmp3 : Outport  Port=3  VectorParamsAs1DForOutWhenUnconnected=off
  wires:
  Multiport Switch2/1 -> Tcmp3/1
  Tc/1 -> Multiport Switch/5, Multiport Switch/6, Multiport Switch1/3, Multiport Switch2/4, Multiport Switch2/2, Multiport Switch1/7
  Multiport Switch1/1 -> Tcmp2/1
  Ta/1 -> Multiport Switch1/2, Multiport Switch1/6, Multiport Switch2/5, Multiport Switch2/7, Multiport Switch/4, Multiport Switch/3
  Multiport Switch/1 -> Tcmp1/1
  Tb/1 -> Multiport Switch/2, Multiport Switch/7, Multiport Switch1/4, Multiport Switch1/5, Multiport Switch2/3, Multiport Switch2/6
  扇区值N/1 -> Multiport Switch/1, Multiport Switch1/1, Multiport Switch2/1

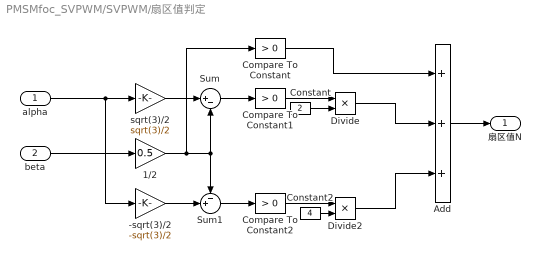
== system PMSMfoc_SVPWM/SVPWM/扇区值判定 ==
  alpha : Inport
  beta : Inport  Port=2
  -sqrt(3)/2 : Gain  Gain=-sqrt(3)/2
  1/2 : Gain  Gain=0.5
  "Add " : Sum  Inputs=+++
  Compare To Constant : simulink/Logic and Bit Operations/Compare To Constant  relop=>  const=0  OutDataTypeStr=boolean
  Compare To Constant1 : simulink/Logic and Bit Operations/Compare To Constant  relop=>  const=0  OutDataTypeStr=boolean
  Compare To Constant2 : simulink/Logic and Bit Operations/Compare To Constant  relop=>  const=0  OutDataTypeStr=boolean
  Constant : Constant  Value=2
  Constant2 : Constant  Value=4
  Divide : Product  Inputs=**
  Divide2 : Product  Inputs=**
  Sum : Sum  Inputs=|+-
  Sum1 : Sum  Inputs=-+|
  sqrt(3)/2 : Gain  Gain=sqrt(3)/2
  扇区值N : Outport  VectorParamsAs1DForOutWhenUnconnected=off
  wires:
  alpha/1 -> sqrt(3)/2/1, -sqrt(3)/2/1
  Constant/1 -> Divide/2
  Divide/1 -> "Add "/2
  Compare To Constant1/1 -> Divide/1
  Compare To Constant/1 -> "Add "/1
  sqrt(3)/2/1 -> Sum/1
  beta/1 -> 1/2/1
  Compare To Constant2/1 -> Divide2/1
  "Add "/1 -> 扇区值N/1
  1/2/1 -> Compare To Constant/1, Sum/2, Sum1/1
  Constant2/1 -> Divide2/2
  Sum1/1 -> Compare To Constant2/1
  -sqrt(3)/2/1 -> Sum1/2
  Sum/1 -> Compare To Constant1/1
  Divide2/1 -> "Add "/3

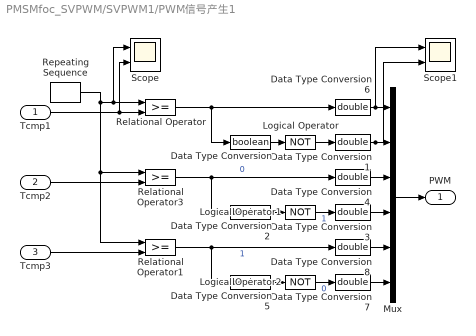
== system PMSMfoc_SVPWM/SVPWM1/PWM信号产生1 ==
  Tcmp1 : Inport
  Tcmp2 : Inport  Port=2
  Tcmp3 : Inport  Port=3
  Data Type Conversion : DataTypeConversion  OutDataTypeStr=boolean
  Data Type Conversion{1,3..4,6..8} (6 alike) : DataTypeConversion  OutDataTypeStr=double
  Data Type Conversion2 : DataTypeConversion  OutDataTypeStr=boolean
  Data Type Conversion5 : DataTypeConversion  OutDataTypeStr=boolean
  Logical Operator : Logic  Operator=NOT  AllPortsSameDT=off  OutDataTypeStr=boolean
  Logical Operator1 : Logic  Operator=NOT  AllPortsSameDT=off  OutDataTypeStr=boolean
  Logical Operator2 : Logic  Operator=NOT  AllPortsSameDT=off  OutDataTypeStr=boolean
  Mux : Mux  Inputs=6
  Relational Operator : RelationalOperator  OutDataTypeStr=boolean  RndMeth=Nearest
  Relational Operator1 : RelationalOperator  OutDataTypeStr=boolean  RndMeth=Nearest
  Relational Operator3 : RelationalOperator  OutDataTypeStr=boolean  RndMeth=Nearest
  Repeating Sequence : simulink/Sources/Repeating Sequence  rep_seq_t=[0 1e-4 2e-4]  rep_seq_y=[0 1.3e-6 0]
  Scope : Scope  NumInputPorts=2
  Scope1 : Scope  NumInputPorts=2
  PWM : Outport  VectorParamsAs1DForOutWhenUnconnected=off
  wires:
  Data Type Conversion/1 -> Logical Operator/1
  Logical Operator/1 -> Data Type Conversion1/1
  Relational Operator/1 -> Data Type Conversion6/1, Data Type Conversion/1
  Logical Operator1/1 -> Data Type Conversion3/1  "1"
  Relational Operator3/1 -> Data Type Conversion4/1, Data Type Conversion2/1  "0"
  Data Type Conversion2/1 -> Logical Operator1/1
  Relational Operator1/1 -> Data Type Conversion8/1, Data Type Conversion5/1  "1"
  Data Type Conversion5/1 -> Logical Operator2/1
  Logical Operator2/1 -> Data Type Conversion7/1  "0"
  Repeating Sequence/1 -> Relational Operator1/1, Relational Operator3/1, Scope/1, Relational Operator/1
  Tcmp1/1 -> Scope/2, Relational Operator/2
  Tcmp2/1 -> Relational Operator3/2
  Tcmp3/1 -> Relational Operator1/2
  Data Type Conversion1/1 -> Scope1/2, Mux/2
  Data Type Conversion4/1 -> Mux/3
  Data Type Conversion3/1 -> Mux/4
  Data Type Conversion8/1 -> Mux/5
  Data Type Conversion7/1 -> Mux/6
  Mux/1 -> PWM/1
  Data Type Conversion6/1 -> Scope1/1, Mux/1

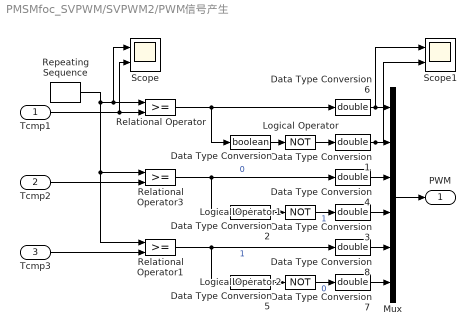
== system PMSMfoc_SVPWM/SVPWM2/PWM信号产生 ==
  Tcmp1 : Inport
  Tcmp2 : Inport  Port=2
  Tcmp3 : Inport  Port=3
  Data Type Conversion : DataTypeConversion  OutDataTypeStr=boolean
  Data Type Conversion{1,3..4,6..8} (6 alike) : DataTypeConversion  OutDataTypeStr=double
  Data Type Conversion2 : DataTypeConversion  OutDataTypeStr=boolean
  Data Type Conversion5 : DataTypeConversion  OutDataTypeStr=boolean
  Logical Operator : Logic  Operator=NOT  AllPortsSameDT=off  OutDataTypeStr=boolean
  Logical Operator1 : Logic  Operator=NOT  AllPortsSameDT=off  OutDataTypeStr=boolean
  Logical Operator2 : Logic  Operator=NOT  AllPortsSameDT=off  OutDataTypeStr=boolean
  Mux : Mux  Inputs=6
  Relational Operator : RelationalOperator  OutDataTypeStr=boolean  RndMeth=Nearest
  Relational Operator1 : RelationalOperator  OutDataTypeStr=boolean  RndMeth=Nearest
  Relational Operator3 : RelationalOperator  OutDataTypeStr=boolean  RndMeth=Nearest
  Repeating Sequence : simulink/Sources/Repeating Sequence  rep_seq_t=[0 1e-4 2e-4]  rep_seq_y=[0 5000 0]
  Scope : Scope  NumInputPorts=2
  Scope1 : Scope  NumInputPorts=2
  PWM : Outport  VectorParamsAs1DForOutWhenUnconnected=off
  wires:
  Data Type Conversion/1 -> Logical Operator/1
  Logical Operator/1 -> Data Type Conversion1/1
  Relational Operator/1 -> Data Type Conversion6/1, Data Type Conversion/1
  Logical Operator1/1 -> Data Type Conversion3/1  "1"
  Relational Operator3/1 -> Data Type Conversion4/1, Data Type Conversion2/1  "0"
  Data Type Conversion2/1 -> Logical Operator1/1
  Relational Operator1/1 -> Data Type Conversion8/1, Data Type Conversion5/1  "1"
  Data Type Conversion5/1 -> Logical Operator2/1
  Logical Operator2/1 -> Data Type Conversion7/1  "0"
  Repeating Sequence/1 -> Relational Operator1/1, Relational Operator3/1, Scope/1, Relational Operator/1
  Tcmp1/1 -> Scope/2, Relational Operator/2
  Tcmp2/1 -> Relational Operator3/2
  Tcmp3/1 -> Relational Operator1/2
  Data Type Conversion1/1 -> Scope1/2, Mux/2
  Data Type Conversion4/1 -> Mux/3
  Data Type Conversion3/1 -> Mux/4
  Data Type Conversion8/1 -> Mux/5
  Data Type Conversion7/1 -> Mux/6
  Mux/1 -> PWM/1
  Data Type Conversion6/1 -> Scope1/1, Mux/1

== matlab function PMSMfoc_SVPWM/SVPWM_Math1/PWM ==
  data: S input double; PWM output double size=[1 6]; t1 input double; t2 input double; time input double; T0 input double
function PWM =fcn(S,t1,t2,time,T0)
% This block supports an embeddable subset of the MATLAB language.
% See the help menu for details. 
%------------------------------普通定义电压---------------------------------
%U0=[0 0 0];U1=[1 0 0];U2=[1 1 0];U3=[0 1 0];
%U4=[0 1 1];U5=[0 0 1];U6=[1 0 1];U7=[1 1 1];
%------------------------由上可得八种电压输出信号控制（每种后面取反）---------
U0=[0 1 0 1 0 1];U1=[1 0 0 1 0 1];U2=[1 0 1 0 0 1];U3=[0 1 1 0 0 1];
U4=[0 1 1 0 1 0];U5=[0 1 0 1 1 0];U6=[1 0 0 1 1 0];U7=[1 0 1 0 1 0];
%----------------------------此处采用二进制定义电压--------------------------
%U0=[0 0 0];U1=[0 0 1];U2=[0 1 0];U3=[0 1 1];
%U4=[1 0 0];U5=[1 0 1];U6=[1 1 0];U7=[1 1 1];
%------------------------由上可得八种电压输出信号控制（每种后面取反）---------
%U0=[0 1 0 1 0 1];U1=[0 1 0 1 1 0];U2=[0 1 1 0 0 1];U3=[0 1 1 0 1 0];
%U4=[1 0 0 1 0 1];U5=[1 0 0 1 1 0];U6=[1 0 1 0 0 1];U7=[1 0 1 0 1 0];
%--------------------------------------------------------------------------
%----------------------为了方便确定扇区切换时间设定的Tx、Ty、Tz---------------
t0=T0-t1-t2;
Ta=t0/4;
Tb=Ta+t1/2;
Tc=Tb+t2/2;
t=rem(time,T0);%t=时间time/周期Ts的余数 即在每个周期内作用的时间轴时间t
G=U0;
%------------------------------扇区编号S------------------------------------
%-------------------------------分割线--------------------------------------
switch (S)
    case 1
        G1=U1;
        G2=U2;
    case 2
        G1=U3;
        G2=U2;
    case 3
        G1=U3;
        G2=U4;
    case 4
        G1=U5;
        G2=U4;
    case 5
        G1=U5;
        G2=U6;
    case 6
        G1=U1;
        G2=U6;
    otherwise
        G1=U0;
        G2=U7;
end
%---------------------------七步分量法--------------------------------------
if (t<Ta)
	G=U0;       
elseif((t>=Ta)&&(t<Tb))
    G=G1;
elseif((t>=Tb)&&(t<Tc))
    G=G2;
elseif((t>=Tc)&&(t<(T0-Tc)))
    G=U7;
elseif((t>=(T0-Tc))&&(t<(T0-Tb)))
    G=G2;
elseif((t>=(T0-Tb))&&(t<(T0-Ta)))
    G=G1;
elseif((t>=(T0-Ta))&&(t<T0))
    G=U0;
end
PWM=G;
end

== matlab function PMSMfoc_SVPWM/SVPWM_Math1/作用时间计算 ==
  data: Us_alfa input; S output; Us_beta input; Udc input; T0 input; t1 output; t2 output
function [S,t1,t2] = fcn(Us_alfa,Us_beta,Udc,T0)
% This block supports an embeddable subset of the MATLAB language.
% See the help menu for details.
%--------------------为了方便推导作用时间做出的设定值------------------------
X=sqrt(3)*T0*Us_beta/Udc;                           
Y=sqrt(3)/2*T0*Us_beta/Udc+3/2*T0*Us_alfa/Udc;     
Z=sqrt(3)/2*T0*Us_beta/Udc-3/2*T0*Us_alfa/Udc;      
%--------------------------------扇区值判断---------------------------------
%Uref1*sqrt(3)
%(Uref1+Uref2)*sqrt(3)
%(Uref1+Uref3)*sqrt(3)
%--------------------------------------------------------------------------
if(Us_beta>0)                                       %Uref1>0
    A=1;
else
    A=0;
end                                                                                                                                                                                                                                                                                                                                                                                                                                                                                                                                                                                                                                                                                                                                                                                                                                                                                                                                                                                                                                                                                                                                                                                                                                                                                   
if((sqrt(3)*Us_alfa-Us_beta)>0)                     %Uref2>0
    B=1;
else
    B=0; 
end
if((-sqrt(3)*Us_alfa-Us_beta)>0)                    %%Uref3>0
    C=1;
else
    C=0;
end
N=A+2*B+4*C;                                        %扇区值N，而不是扇区编号！！！！！！！
%--------------------------------------------------------------------------
%-----------------------------------分割线----------------------------------

%-----------------------------矢量作用时间计算-------------------------------
%--------------------------------S为扇区编号-------------------------------
switch(N)
    case 1
        S=2;%----------------------扇区编号S---------------------------
        t1=Z; 
        t2=Y; 
    case 2
        S=6;
        t1=Y; 
        t2=-X;
    case 3
        S=1;
        t1=-Z; 
        t2=X;
    case 4
        S=4;
        t1=-X; 
        t2=Z;
    case 5
        S=3;
        t1=X; 
        t2=-Y;
    case 6
        S=5;
        t1=-Y; 
        t2=-Z;
    otherwise
        S=1;
        t1=0; 
        t2=0;        
end
%--------------------------------------------------------------------------
%-----------------------------是否需要调制判断------------------------------
if((t1+t2)>T0)
    t11=t1*T0/(t1+t2);
    t21=t2*T0/(t1+t2);
    t1=t11;
    t2=t21;
    t0=0;
else
t0=T0-t1-t2;
end
%--------------------------------------------------------------------------
